simulink model "FG_traj_fast"  (Simulink 8.1)
settings: Solver=FixedStepDiscrete  StartTime=0.0  StopTime=inf  FixedStep=Ts  RelTol=1e-3
PreLoadFcn:
  | load_waypoints
values from neighbouring files (symbols this model uses):
  g = 9.8065    [kostas_malakies.mat]    (also in kostas_malakies2.mat; load_PMModel.m = 9.81; main.m; main_last.m)
  pitch_cmd2pitch_1stOrd = 1.42468924998    [kostas_malakies.mat]    (also in kostas_malakies2.mat)
  roll_cmd2roll_1stOrd = 1.38101661575    [kostas_malakies.mat]    (also in kostas_malakies2.mat)
  thrust_cmd2thrust_0thOrd = 0.876575459522    [kostas_malakies.mat]    (also in kostas_malakies2.mat)
  THRUST_CMD_GAIN = -0.0835    [kostas_malakies.mat]    (also in kostas_malakies2.mat; load_PMModel.m)
  yaw_cmd2yaw_1stOrd = 2.01792090263    [kostas_malakies.mat]    (also in kostas_malakies2.mat)
libraries: Hquad_control_LIB_MPC x4, simulink x1
settings Model: Creator=janosch  LastModifiedBy=burrimi  SimulationMode=external
settings DataIOCC: SaveOutput=off  SaveTime=off
settings OptimizationCC: OptimizeModelRefInitCode=on  LifeSpan=Inf
settings DebuggingCC: ParameterPrecisionLossMsg=none
settings HardwareCC: ProdIntDivRoundTo=Zero  ProdEndianess=LittleEndian  ProdHWDeviceType=Intel Pentium
settings RTWCC: SystemTargetFile=ert.tlc  TemplateMakefile=ert_default_tmf  Description=Embedded Coder  ProcessScript=ert_make_rtw_hook  CustomHeaderCode=#include <math.h>  TargetLang=C++  RTWCompilerOptimization=On
settings CodeAppCC: IgnoreCustomStorageClasses=off  CustomSymbolStrType=$N$R$M  InternalIdentifier=Classic
settings ERTTargetCC: CodeReplacementLibrary=ANSI_C  MultiwordLength=2048  GenerateSampleERTMain=on  SupportNonInlinedSFcns=on  ExtMode=on  ERTCustomFileTemplate=example_file_process.tlc  ConvertIfToSwitch=off  SuppressUnreachableDefaultCases=off
settings ConfigurationSet: Description=SimMechanics 2G

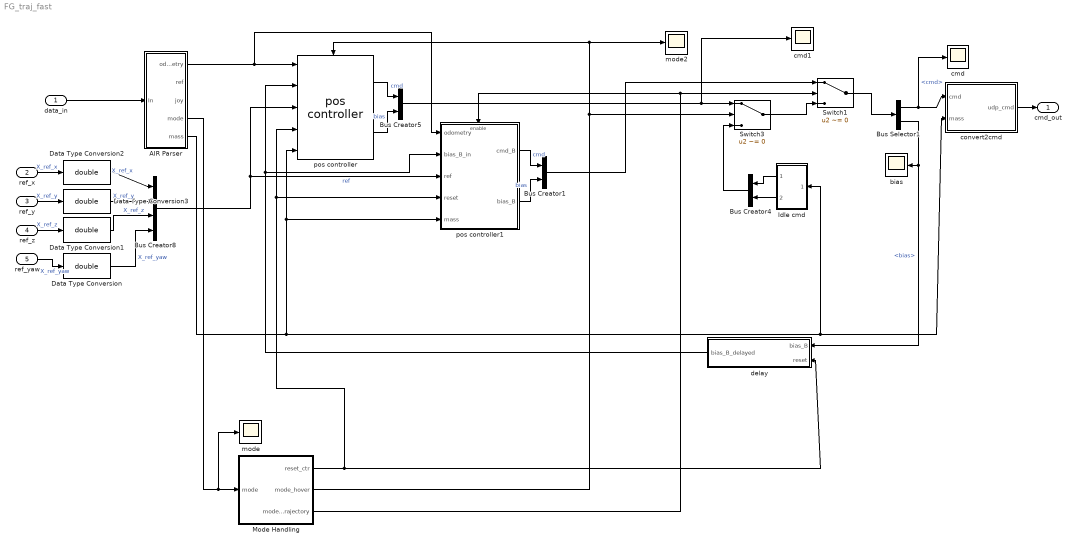
== system FG_traj_fast ==
  data_in : Inport  OutDataTypeStr=single  PortDimensions=30
  ref_x : Inport  Port=2  OutDataTypeStr=single  PortDimensions=93
  ref_y : Inport  Port=3  OutDataTypeStr=single  PortDimensions=93
  ref_z : Inport  Port=4  OutDataTypeStr=single  PortDimensions=62
  ref_yaw : Inport  Port=5  OutDataTypeStr=single  PortDimensions=62
  AIR Parser : Subsystem
  Bus Creator1 : BusCreator  Inputs=2
  Bus Creator4 : BusCreator  Inputs=2
  Bus Creator5 : BusCreator  Inputs=2
  Bus Creator8 : BusCreator
  Bus Selector1 : BusSelector  OutputSignals=cmd,bias
  Data Type Conversion{,1..3} (4 alike) : DataTypeConversion  OutDataTypeStr=double
  Idle cmd : Subsystem
  Mode Handling : Subsystem
  Switch1 : Switch  Criteria=u2 ~= 0
  Switch3 : Switch  Criteria=u2 ~= 0
  bias : Scope
      settings: TickLabels=on  TimeRange=40  YMin=-0.3  YMax=0.075  SaveName=ScopeData9
  cmd : Scope
      settings: YMin=-0.5  YMax=7  SaveName=ScopeData4
  cmd1 : Scope
      settings: YMin=-0.5  YMax=7  SaveName=ScopeData15
  convert2cmd : Subsystem
  delay : Subsystem
  mode : Scope
      settings: YMin=0  YMax=6  SaveName=ScopeData6
  mode2 : Scope
      settings: YMin=0  YMax=6  SaveName=ScopeData14
  pos controller : Hquad_control_LIB_MPC/pos controller
  pos controller1 : Subsystem  AncestorBlock=Hquad_control_LIB_MPC/pos controller
  cmd_out : Outport  PortDimensions=4
  wires:
  Mode Handling/1(reset_ctr) -> delay/2(reset), pos controller1/4(reset), pos controller/4
  Mode Handling/2(mode_hover) -> Switch3/2, mode2/1, pos controller/Enable
  AIR Parser/4(mode) -> mode/1, Mode Handling/1(mode)
  Bus Creator5/1 -> Switch3/1, cmd1/1
  pos controller/1 -> Bus Creator5/1  "cmd"
  pos controller/2 -> Bus Creator5/2  "bias"
  Bus Selector1/1 -> convert2cmd/1(cmd), cmd/1  "<cmd>"
  Bus Selector1/2 -> bias/1, delay/1(bias_B)  "<bias>"
  delay/1(bias_B_delayed) -> pos controller1/2(bias_B_in), pos controller/2
  convert2cmd/1(udp_cmd) -> cmd_out/1
  data_in/1 -> AIR Parser/1(In)
  Idle cmd/1(cmd) -> Bus Creator4/1
  Idle cmd/2(bias) -> Bus Creator4/2
  Bus Creator4/1 -> Switch3/3
  AIR Parser/1(odometry) -> pos controller1/1(odometry), pos controller/1
  ref_x/1 -> Data Type Conversion2/1  "X_ref_x"
  ref_y/1 -> Data Type Conversion3/1  "X_ref_y"
  ref_z/1 -> Data Type Conversion1/1  "X_ref_z"
  ref_yaw/1 -> Data Type Conversion/1  "X_ref_yaw"
  Data Type Conversion/1 -> Bus Creator8/4  "X_ref_yaw"
  Data Type Conversion1/1 -> Bus Creator8/3  "X_ref_z"
  Data Type Conversion2/1 -> Bus Creator8/1  "X_ref_x"
  Data Type Conversion3/1 -> Bus Creator8/2  "X_ref_y"
  Switch3/1 -> Switch1/3
  Switch1/1 -> Bus Selector1/1
  Mode Handling/3(mode_trajectory) -> pos controller1/Enable, Switch1/2
  AIR Parser/5(mass) -> Idle cmd/1(mass), convert2cmd/2(mass), pos controller1/5(mass), pos controller/5
  Bus Creator8/1 -> pos controller1/3(ref), pos controller/3  "ref"
  Bus Creator1/1 -> Switch1/1
  pos controller1/1(cmd_B) -> Bus Creator1/1  "cmd"
  pos controller1/2(bias_B) -> Bus Creator1/2  "bias"

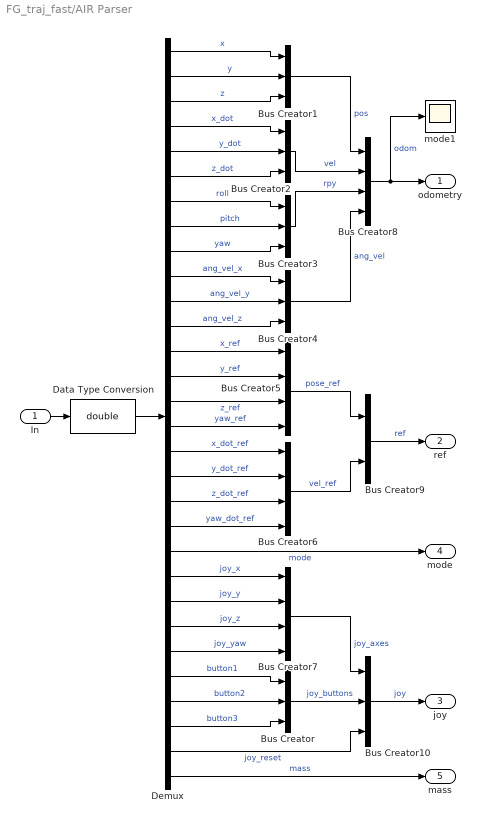
== system FG_traj_fast/AIR Parser ==
  In : Inport
  Bus Creator{,1..4,10} (6 alike) : BusCreator  Inputs=3
  Bus Creator{5..8} (4 alike) : BusCreator
  Bus Creator9 : BusCreator  Inputs=2
  Data Type Conversion : DataTypeConversion  OutDataTypeStr=double
  Demux : Demux  Outputs=30
  mode1 : Scope
      settings: YMin=0  YMax=6  SaveName=ScopeData7
  odometry : Outport
  ref : Outport  Port=2
  joy : Outport  Port=3
  mode : Outport  Port=4
  mass : Outport  Port=5
  wires:
  In/1 -> Data Type Conversion/1
  Data Type Conversion/1 -> Demux/1
  Demux/1 -> Bus Creator1/1  "x"
  Demux/7 -> Bus Creator3/1  "roll"
  Demux/8 -> Bus Creator3/2  "pitch"
  Demux/9 -> Bus Creator3/3  "yaw"
  Demux/15 -> Bus Creator5/3  "z_ref"
  Demux/14 -> Bus Creator5/2  "y_ref"
  Demux/13 -> Bus Creator5/1  "x_ref"
  Demux/16 -> Bus Creator5/4  "yaw_ref"
  Demux/2 -> Bus Creator1/2  "y"
  Demux/3 -> Bus Creator1/3  "z"
  Demux/4 -> Bus Creator2/1  "x_dot"
  Demux/5 -> Bus Creator2/2  "y_dot"
  Demux/6 -> Bus Creator2/3  "z_dot"
  Demux/19 -> Bus Creator6/3  "z_dot_ref"
  Demux/18 -> Bus Creator6/2  "y_dot_ref"
  Demux/17 -> Bus Creator6/1  "x_dot_ref"
  Demux/20 -> Bus Creator6/4  "yaw_dot_ref"
  Demux/12 -> Bus Creator4/3  "ang_vel_z"
  Demux/11 -> Bus Creator4/2  "ang_vel_y"
  Demux/10 -> Bus Creator4/1  "ang_vel_x"
  Demux/21 -> mode/1  "mode"
  Bus Creator5/1 -> Bus Creator9/1  "pose_ref"
  Bus Creator6/1 -> Bus Creator9/2  "vel_ref"
  Demux/22 -> Bus Creator7/1  "joy_x"
  Demux/23 -> Bus Creator7/2  "joy_y"
  Demux/24 -> Bus Creator7/3  "joy_z"
  Demux/25 -> Bus Creator7/4  "joy_yaw"
  Bus Creator7/1 -> Bus Creator10/1  "joy_axes"
  Demux/26 -> Bus Creator/1  "button1"
  Demux/28 -> Bus Creator/3  "button3"
  Demux/27 -> Bus Creator/2  "button2"
  Bus Creator/1 -> Bus Creator10/2  "joy_buttons"
  Bus Creator4/1 -> Bus Creator8/4  "ang_vel"
  Bus Creator3/1 -> Bus Creator8/3  "rpy"
  Bus Creator2/1 -> Bus Creator8/2  "vel"
  Bus Creator1/1 -> Bus Creator8/1  "pos"
  Demux/29 -> Bus Creator10/3  "joy_reset"
  Bus Creator10/1 -> joy/1  "joy"
  Bus Creator9/1 -> ref/1  "ref"
  Bus Creator8/1 -> odometry/1, mode1/1  "odom"
  Demux/30 -> mass/1  "mass"

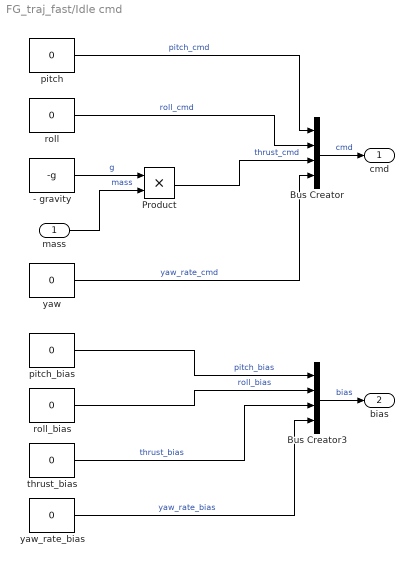
== system FG_traj_fast/Idle cmd ==
  mass : Inport  OutDataTypeStr=double
  - gravity : Constant  Value=-g
  Bus Creator : BusCreator
  Bus Creator3 : BusCreator
  Product : Product  RndMeth=Zero
  pitch : Constant  Value=0
  pitch_bias : Constant  Value=0
  roll : Constant  Value=0
  roll_bias : Constant  Value=0
  thrust_bias : Constant  Value=0
  yaw : Constant  Value=0
  yaw_rate_bias : Constant  Value=0
  cmd : Outport
  bias : Outport  Port=2
  wires:
  roll/1 -> Bus Creator/2  "roll_cmd"
  pitch/1 -> Bus Creator/1  "pitch_cmd"
  Bus Creator/1 -> cmd/1  "cmd"
  yaw/1 -> Bus Creator/4  "yaw_rate_cmd"
  pitch_bias/1 -> Bus Creator3/1  "pitch_bias"
  roll_bias/1 -> Bus Creator3/2  "roll_bias"
  thrust_bias/1 -> Bus Creator3/3  "thrust_bias"
  yaw_rate_bias/1 -> Bus Creator3/4  "yaw_rate_bias"
  Bus Creator3/1 -> bias/1  "bias"
  - gravity/1 -> Product/1  "g"
  Product/1 -> Bus Creator/3  "thrust_cmd"
  mass/1 -> Product/2  "mass"

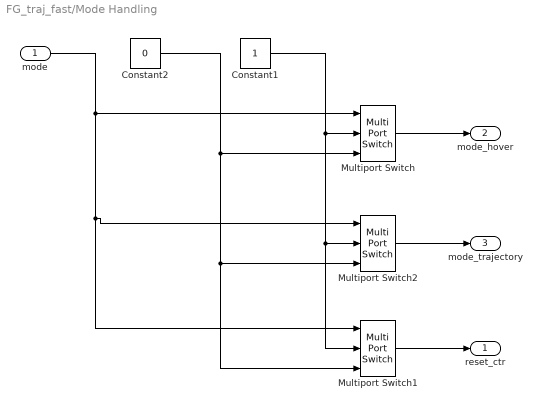
== system FG_traj_fast/Mode Handling ==
  mode : Inport
  Constant1 : Constant
  Constant2 : Constant  Value=0
  Multiport Switch : MultiPortSwitch  DataPortOrder=Specify indices  Inputs=2  DataPortIndices={[1,2,3],0}
  Multiport Switch1 : MultiPortSwitch  DataPortOrder=Specify indices  Inputs=2  DataPortIndices={[10],0}
  Multiport Switch2 : MultiPortSwitch  DataPortOrder=Specify indices  Inputs=2  DataPortIndices={[4],0}
  reset_ctr : Outport
  mode_hover : Outport  Port=2
  mode_trajectory : Outport  Port=3
  wires:
  Constant1/1 -> Multiport Switch/2, Multiport Switch1/2, Multiport Switch2/2
  Constant2/1 -> Multiport Switch/3, Multiport Switch1/3, Multiport Switch2/3
  Multiport Switch1/1 -> reset_ctr/1
  mode/1 -> Multiport Switch/1, Multiport Switch1/1, Multiport Switch2/1
  Multiport Switch/1 -> mode_hover/1
  Multiport Switch2/1 -> mode_trajectory/1

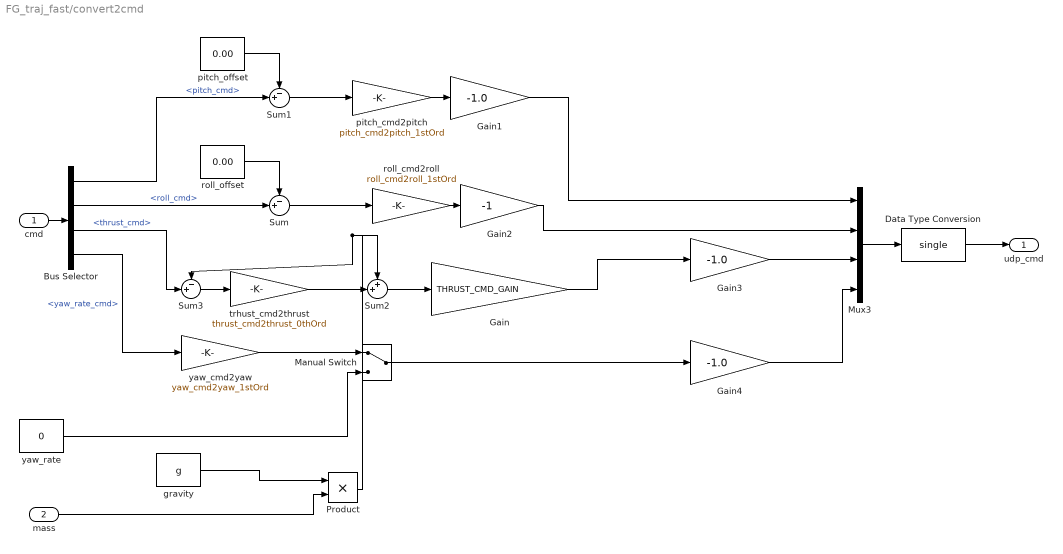
== system FG_traj_fast/convert2cmd ==
  cmd : Inport
  mass : Inport  Port=2
  Bus Selector : BusSelector  OutputSignals=pitch_cmd,roll_cmd,thrust_cmd,yaw_rate_cmd
  Data Type Conversion : DataTypeConversion  OutDataTypeStr=single
  Gain : Gain  Gain=THRUST_CMD_GAIN
  Gain1 : Gain  Gain=-1.0
  Gain2 : Gain  Gain=-1
  Gain3 : Gain  Gain=-1.0
  Gain4 : Gain  Gain=-1.0
  Manual Switch : ManualSwitch
  Mux3 : Mux
  Product : Product  RndMeth=Zero
  Sum : Sum  Inputs=-+|
  Sum1 : Sum  Inputs=-+|
  Sum2 : Sum  Inputs=++|
  Sum3 : Sum  Inputs=-+|
  gravity : Constant  Value=g
  pitch_cmd2pitch : Gain  Gain=pitch_cmd2pitch_1stOrd
  pitch_offset : Constant  Value=0.00
  roll_cmd2roll : Gain  Gain=roll_cmd2roll_1stOrd
  roll_offset : Constant  Value=0.00
  trhust_cmd2thrust : Gain  Gain=thrust_cmd2thrust_0thOrd
  yaw_cmd2yaw : Gain  Gain=yaw_cmd2yaw_1stOrd
  yaw_rate : Constant  Value=0
  udp_cmd : Outport
  wires:
  pitch_cmd2pitch/1 -> Gain1/1
  Bus Selector/2 -> Sum/2  "<roll_cmd>"
  Sum/1 -> roll_cmd2roll/1
  roll_offset/1 -> Sum/1
  Gain4/1 -> Mux3/4
  Gain3/1 -> Mux3/3
  Gain2/1 -> Mux3/2
  Gain/1 -> Gain3/1
  Gain1/1 -> Mux3/1
  pitch_offset/1 -> Sum1/1
  Sum1/1 -> pitch_cmd2pitch/1
  Mux3/1 -> Data Type Conversion/1
  Data Type Conversion/1 -> udp_cmd/1
  Product/1 -> Sum2/1, Sum3/1
  Sum2/1 -> Gain/1
  Manual Switch/1 -> Gain4/1
  yaw_rate/1 -> Manual Switch/2
  cmd/1 -> Bus Selector/1
  Bus Selector/1 -> Sum1/2  "<pitch_cmd>"
  yaw_cmd2yaw/1 -> Manual Switch/1
  trhust_cmd2thrust/1 -> Sum2/2
  roll_cmd2roll/1 -> Gain2/1
  Bus Selector/3 -> Sum3/2  "<thrust_cmd>"
  Sum3/1 -> trhust_cmd2thrust/1
  Bus Selector/4 -> yaw_cmd2yaw/1  "<yaw_rate_cmd>"
  gravity/1 -> Product/1
  mass/1 -> Product/2

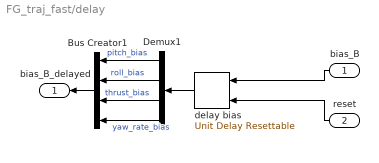
== system FG_traj_fast/delay ==
  bias_B : Inport
  reset : Inport  Port=2
  Bus Creator1 : BusCreator
  Demux1 : Demux
  delay bias : simulink/Additional Math & Discrete/Additional Discrete/Unit Delay Resettable  vinit=0.0  tsamp=-1
  bias_B_delayed : Outport
  wires:
  Demux1/1 -> Bus Creator1/1  "pitch_bias"
  Demux1/2 -> Bus Creator1/2  "roll_bias"
  Demux1/3 -> Bus Creator1/3  "thrust_bias"
  Demux1/4 -> Bus Creator1/4  "yaw_rate_bias"
  delay bias/1 -> Demux1/1
  bias_B/1 -> delay bias/1
  reset/1 -> delay bias/2
  Bus Creator1/1 -> bias_B_delayed/1

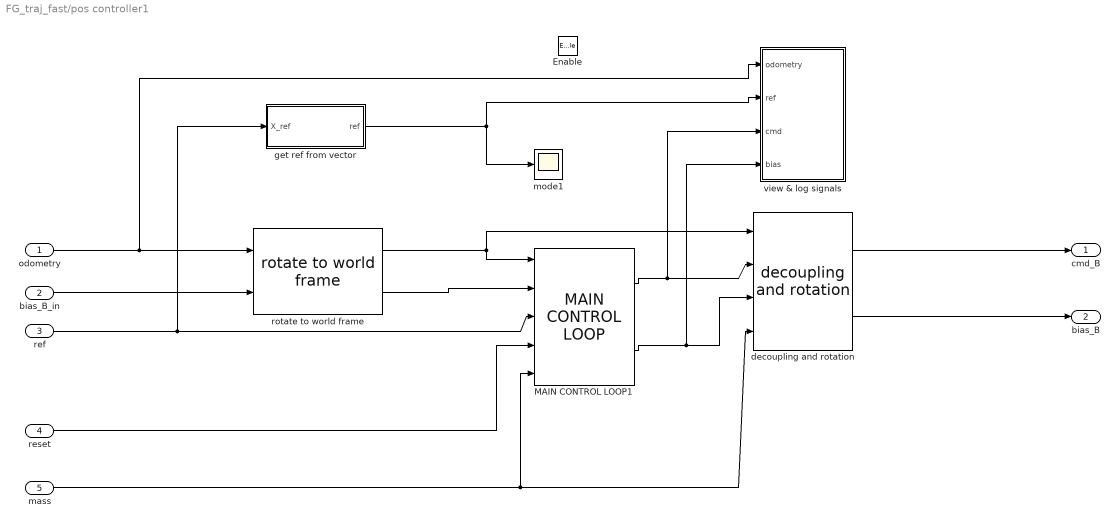
== system FG_traj_fast/pos controller1 ==
  odometry : Inport
  bias_B_in : Inport  Port=2
  ref : Inport  Port=3
  reset : Inport  Port=4
  mass : Inport  Port=5
  Enable : EnablePort  StatesWhenEnabling=reset
  MAIN CONTROL LOOP1 : Hquad_control_LIB_MPC/MAIN CONTROL LOOP  Priority=2
  decoupling and rotation : Hquad_control_LIB_MPC/decoupling and rotation  Priority=3
  get ref from vector : Subsystem
  mode1 : Scope
      settings: YMin=0  YMax=6  SaveName=ScopeData12
  rotate to world frame : Hquad_control_LIB_MPC/rotate to world frame  Priority=1
  view & log signals : Subsystem  AncestorBlock=Hquad_control_LIB_MPC/view & log signals
  cmd_B : Outport
  bias_B : Outport  Port=2
  wires:
  MAIN CONTROL LOOP1/1 -> decoupling and rotation/2, view & log signals/3(cmd)
  odometry/1 -> rotate to world frame/1, view & log signals/1(odometry)
  reset/1 -> MAIN CONTROL LOOP1/4
  ref/1 -> get ref from vector/1(X_ref), MAIN CONTROL LOOP1/3
  get ref from vector/1(ref) -> view & log signals/2(ref), mode1/1
  rotate to world frame/1 -> MAIN CONTROL LOOP1/1, decoupling and rotation/1
  MAIN CONTROL LOOP1/2 -> decoupling and rotation/3, view & log signals/4(bias)
  decoupling and rotation/1 -> cmd_B/1
  decoupling and rotation/2 -> bias_B/1
  rotate to world frame/2 -> MAIN CONTROL LOOP1/2
  bias_B_in/1 -> rotate to world frame/2
  mass/1 -> MAIN CONTROL LOOP1/5, decoupling and rotation/4

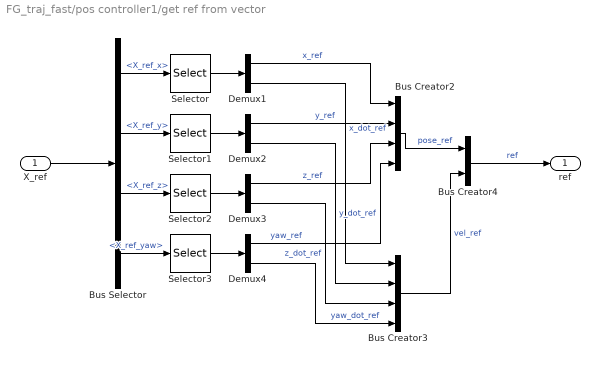
== system FG_traj_fast/pos controller1/get ref from vector ==
  X_ref : Inport
  Bus Creator2 : BusCreator
  Bus Creator3 : BusCreator
  Bus Creator4 : BusCreator  Inputs=2
  Bus Selector : BusSelector  OutputSignals=X_ref_x,X_ref_y,X_ref_z,X_ref_yaw
  Demux{1..4} (4 alike) : Demux  Outputs=2
  Selector{,1..3} (4 alike) : Selector  IndexOptions=Index vector (dialog)  Indices=[1 2]  OutputSizes=1
  ref : Outport
  wires:
  X_ref/1 -> Bus Selector/1
  Bus Selector/1 -> Selector/1  "<X_ref_x>"
  Bus Selector/4 -> Selector3/1  "<X_ref_yaw>"
  Bus Selector/3 -> Selector2/1  "<X_ref_z>"
  Bus Selector/2 -> Selector1/1  "<X_ref_y>"
  Selector/1 -> Demux1/1
  Selector3/1 -> Demux4/1
  Selector2/1 -> Demux3/1
  Selector1/1 -> Demux2/1
  Bus Creator2/1 -> Bus Creator4/1  "pose_ref"
  Bus Creator3/1 -> Bus Creator4/2  "vel_ref"
  Bus Creator4/1 -> ref/1  "ref"
  Demux1/1 -> Bus Creator2/1  "x_ref"
  Demux2/1 -> Bus Creator2/2  "y_ref"
  Demux3/1 -> Bus Creator2/3  "z_ref"
  Demux4/1 -> Bus Creator2/4  "yaw_ref"
  Demux1/2 -> Bus Creator3/1  "x_dot_ref"
  Demux2/2 -> Bus Creator3/2  "y_dot_ref"
  Demux3/2 -> Bus Creator3/3  "z_dot_ref"
  Demux4/2 -> Bus Creator3/4  "yaw_dot_ref"

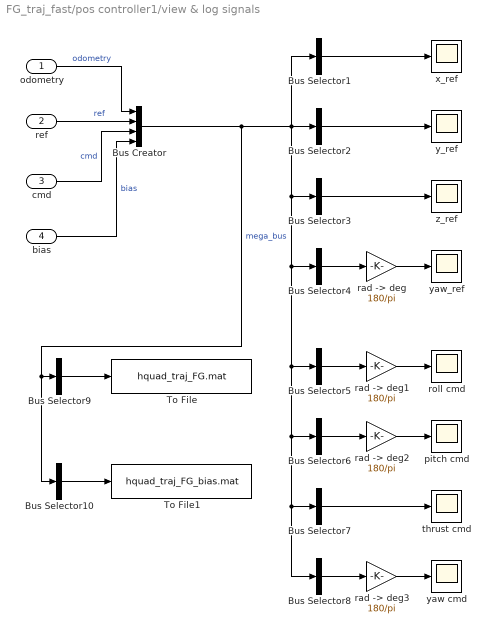
== system FG_traj_fast/pos controller1/view & log signals ==
  odometry : Inport
  ref : Inport  Port=2
  cmd : Inport  Port=3
  bias : Inport  Port=4
  Bus Creator : BusCreator
  Bus Selector1 : BusSelector  OutputSignals=odometry.pos.x,odometry.vel.x_dot,ref.pose_ref.x_ref,ref.vel_ref.x_dot_ref  OutputAsBus=on
  Bus Selector10 : BusSelector  OutputSignals=bias.pitch_bias,bias.roll_bias,bias.thrust_bias,bias.yaw_rate_bias  OutputAsBus=on
  Bus Selector2 : BusSelector  OutputSignals=odometry.pos.y,odometry.vel.y_dot,ref.pose_ref.y_ref,ref.vel_ref.y_dot_ref  OutputAsBus=on
  Bus Selector3 : BusSelector  OutputSignals=odometry.pos.z,odometry.vel.z_dot,ref.pose_ref.z_ref,ref.vel_ref.z_dot_ref  OutputAsBus=on
  Bus Selector4 : BusSelector  OutputSignals=odometry.rpy.yaw,odometry.ang_vel.ang_vel_z,ref.pose_ref.yaw_ref,ref.vel_ref.yaw_dot_ref  OutputAsBus=on
  Bus Selector5 : BusSelector  OutputSignals=odometry.rpy.roll,odometry.ang_vel.ang_vel_x,cmd.roll_cmd  OutputAsBus=on
  Bus Selector6 : BusSelector  OutputSignals=odometry.rpy.pitch,odometry.ang_vel.ang_vel_y,cmd.pitch_cmd  OutputAsBus=on
  Bus Selector7 : BusSelector  OutputSignals=odometry.pos.z,ref.pose_ref.z_ref,cmd.thrust_cmd  OutputAsBus=on
  Bus Selector8 : BusSelector  OutputSignals=odometry.rpy.yaw,odometry.ang_vel.ang_vel_z,cmd.yaw_rate_cmd  OutputAsBus=on
  Bus Selector9 : BusSelector  OutputSignals=odometry.pos.x,odometry.vel.x_dot,odometry.rpy.pitch,ref.pose_ref.x_ref,cmd.pitch_cmd,odometry.pos.y,odometry.vel.y_dot,odometry.rpy.roll,ref.pose_ref.y_ref,cmd.roll_cmd,odometry.pos.z,odometry.vel.z_dot,ref.pose_ref.z_ref,cmd.thrust_cmd,odometry.rpy.yaw,odometry.ang_vel.ang_vel_z,ref.pose_ref.yaw_ref,cmd.yaw_rate_cmd  OutputAsBus=on
  To File : ToFile  Filename=hquad_traj_FG.mat  MatrixName=hquad_pos_FG
  To File1 : ToFile  Filename=hquad_traj_FG_bias.mat  MatrixName=hquad_pos_FG_bias
  pitch cmd : Scope
      settings: YMin=-15  YMax=15  SaveName=ScopeData2
  rad -> deg{,1..3} (4 alike) : Gain  Gain=180/pi
  roll cmd : Scope
      settings: YMin=-100  YMax=100
  thrust cmd : Scope
      settings: YMin=-3  YMax=3  SaveName=ScopeData11
  x_ref : Scope
      settings: YMin=-1.5  YMax=1.5  SaveName=ScopeData3
  y_ref : Scope
      settings: TimeRange=40  YMin=-0.75  YMax=2.75
  yaw cmd : Scope
      settings: YMin=-60  YMax=60  SaveName=ScopeData10
  yaw_ref : Scope
      settings: TimeRange=39.996  YMin=-190  YMax=190  SaveName=ScopeData8
  z_ref : Scope
      settings: TimeRange=40  YMin=-21  YMax=1  SaveName=ScopeData5
  wires:
  bias/1 -> Bus Creator/4  "bias"
  Bus Selector8/1 -> "rad -> deg3"/1
  Bus Selector6/1 -> "rad -> deg2"/1
  Bus Selector5/1 -> "rad -> deg1"/1
  Bus Selector7/1 -> thrust cmd/1
  Bus Selector4/1 -> "rad -> deg"/1
  Bus Selector3/1 -> z_ref/1
  Bus Selector2/1 -> y_ref/1
  Bus Selector1/1 -> x_ref/1
  Bus Creator/1 -> Bus Selector8/1, Bus Selector7/1, Bus Selector6/1, Bus Selector5/1, Bus Selector4/1, Bus Selector3/1, Bus Selector2/1, Bus Selector1/1, Bus Selector10/1, Bus Selector9/1  "mega_bus"
  cmd/1 -> Bus Creator/3  "cmd"
  ref/1 -> Bus Creator/2  "ref"
  odometry/1 -> Bus Creator/1  "odometry"
  "rad -> deg3"/1 -> yaw cmd/1
  "rad -> deg2"/1 -> pitch cmd/1
  "rad -> deg1"/1 -> roll cmd/1
  "rad -> deg"/1 -> yaw_ref/1
  Bus Selector10/1 -> To File1/1
  Bus Selector9/1 -> To File/1
